simulink model "ADRC_playground"  (R2024b)
settings: Solver=FixedStepAuto  StartTime=0.0  StopTime=10.0  FixedStep=h  RelTol=1e-5
values from neighbouring files (symbols this model uses):
  a1 = 2    [ADRC_playground.m]    (also in ADRC_playground_vars.m)
  a2 = 3    [ADRC_playground.m]    (also in ADRC_playground_vars.m)
  b = 0.2    [ADRC_playground_vars.m]    (also in LADRC_ct_vars.m = [zeros(N-1, 1))
  b0 = 0.4    [ADRC_playground_vars.m]    (also in LADRC_ct_vars.m = 0.75)
  beta1 = 1    [ADRC_playground_vars.m]
  beta2 = 1 / (2*h^0.5)    (= 5)    [ADRC_playground_vars.m]
  beta3 = 2 / (5^2 * h^1.2)    (= 20.0950914521)    [ADRC_playground_vars.m]
  c = 1    [ADRC_playground_vars.m]
  h = 0.01    [ADRC_playground_vars.m]
  r = 5    [ADRC_playground_vars.m]
undefined symbols (not defined in the file or in its folder): DiscIntNeverNeededParam
settings Model: Creator=Henrik  LastModifiedBy=Henrik

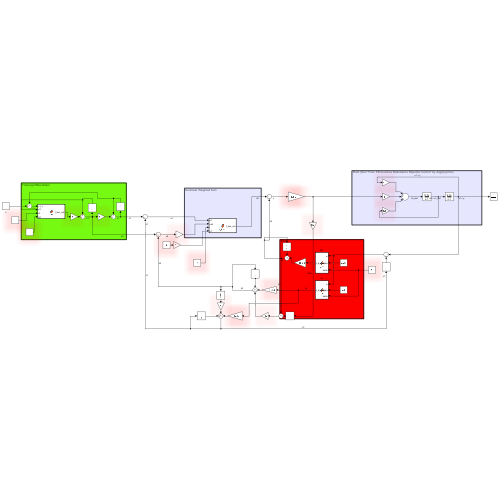
[thumbnail: Simulink's stored preview of the top-level diagram]
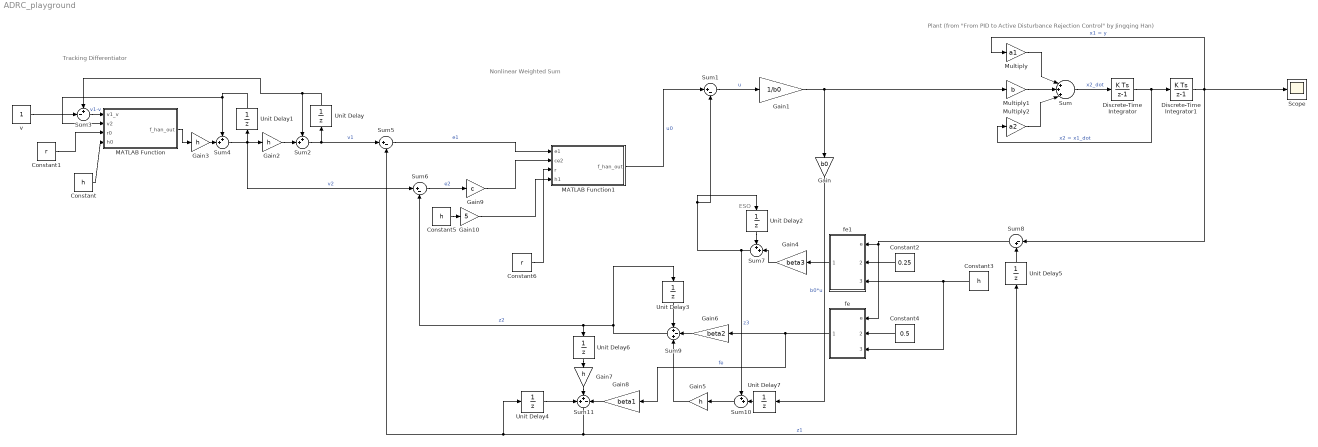
== system ADRC_playground ==
  note: Tracking Differentiator
  note: Nonlinear Weighted Sum
  note: ESO
  note: Plant (from "From PID to Active Disturbance Rejection Control" by Jingqing Han)
  Constant : Constant  Value=h
  Constant1 : Constant  Value=r
  Constant2 : Constant  Value=0.25
  Constant3 : Constant  Value=h
  Constant4 : Constant  Value=0.5
  Constant5 : Constant  Value=h
  Constant6 : Constant  Value=r
  Discrete-Time Integrator : DiscreteIntegrator  SampleTime=-1  ICPrevOutput=DiscIntNeverNeededParam  ICPrevScaledInput=DiscIntNeverNeededParam
  Discrete-Time Integrator1 : DiscreteIntegrator  SampleTime=-1  ICPrevOutput=DiscIntNeverNeededParam  ICPrevScaledInput=DiscIntNeverNeededParam
  Gain : Gain  Gain=b0
  Gain1 : Gain  Gain=1/b0
  Gain10 : Gain  Gain=5
  Gain{2..3,5,7} (4 alike) : Gain  Gain=h
  Gain4 : Gain  Gain=beta3
  Gain6 : Gain  Gain=beta2
  Gain8 : Gain  Gain=beta1
  Gain9 : Gain  Gain=c
  MATLAB Function : MATLAB Function  TreatAsAtomicUnit=on
  MATLAB Function1 : MATLAB Function  TreatAsAtomicUnit=on
  Multiply : Gain  Gain=a1
  Multiply1 : Gain  Gain=b
  Multiply2 : Gain  Gain=a2
  Scope : Scope
  Sum : Sum  Inputs=|+++|
  Sum1 : Sum  Inputs=|+-
  Sum{2,4,7,10} (4 alike) : Sum  Inputs=++|
  Sum11 : Sum  Inputs=++-
  Sum3 : Sum  Inputs=+-|
  Sum5 : Sum  Inputs=|+-
  Sum6 : Sum  Inputs=|+-
  Sum8 : Sum  Inputs=|-+
  Sum9 : Sum  Inputs=+-+
  Unit Delay{,1..7} (8 alike) : UnitDelay  SampleTime=-1  HasFrameUpgradeWarning=on
  fe : MATLAB Function  TreatAsAtomicUnit=on
  fe1 : MATLAB Function  TreatAsAtomicUnit=on
  v : Constant
  wires:
  Multiply2/1 -> Sum/3
  Multiply1/1 -> Sum/2
  Multiply/1 -> Sum/1
  Sum/1 -> Discrete-Time Integrator/1  "x2_dot"
  Discrete-Time Integrator/1 -> Discrete-Time Integrator1/1, Multiply2/1  "x2 = x1_dot"
  Discrete-Time Integrator1/1 -> Scope/1, Sum8/1, Multiply/1  "x1 = y"
  Sum1/1 -> Gain1/1  "u"
  Gain/1 -> Unit Delay7/1  "b0*u"
  Gain1/1 -> Multiply1/1, Gain/1
  Sum7/1 -> Unit Delay2/1, Sum1/2, Sum10/1  "z3"
  MATLAB Function1/1(f_han_out) -> Sum1/1  "u0"
  v/1 -> Sum3/2
  Sum3/1 -> MATLAB Function/1(v1_v)  "v1-v"
  Sum2/1 -> Sum5/1, Unit Delay/1  "v1"
  Unit Delay/1 -> Sum3/1, Sum2/1
  Constant/1 -> MATLAB Function/4(h0)
  Sum4/1 -> Sum6/1, Gain2/1, Unit Delay1/1  "v2"
  Gain2/1 -> Sum2/2
  Unit Delay1/1 -> MATLAB Function/2(v2), Sum4/1
  Gain3/1 -> Sum4/2
  MATLAB Function/1(f_han_out) -> Gain3/1
  Constant1/1 -> MATLAB Function/3(r0)
  Sum9/1 -> Unit Delay6/1, Sum6/2, Unit Delay3/1  "z2"
  fe1/1(f_al_out) -> Gain4/1
  Gain4/1 -> Sum7/2
  Unit Delay2/1 -> Sum7/1
  Sum5/1 -> MATLAB Function1/1(e1)  "e1"
  Sum8/1 -> fe1/1(e), fe/1(e)
  Constant2/1 -> fe1/2(alpha)
  Constant3/1 -> fe1/3(delta), fe/3(delta)
  Unit Delay3/1 -> Sum9/1
  Constant4/1 -> fe/2(alpha)
  fe/1(f_al_out) -> Gain8/1, Gain6/1  "fe"
  Gain6/1 -> Sum9/2
  Sum10/1 -> Gain5/1
  Gain5/1 -> Sum9/3
  Unit Delay4/1 -> Sum11/1
  Sum11/1 -> Unit Delay5/1, Sum5/2, Unit Delay4/1  "z1"
  Gain7/1 -> Sum11/2
  Gain8/1 -> Sum11/3
  Sum6/1 -> Gain9/1  "e2"
  Gain9/1 -> MATLAB Function1/2(ce2)
  Constant5/1 -> Gain10/1
  Gain10/1 -> MATLAB Function1/4(h1)
  Constant6/1 -> MATLAB Function1/3(r)
  Unit Delay5/1 -> Sum8/2
  Unit Delay6/1 -> Gain7/1
  Unit Delay7/1 -> Sum10/2

== matlab function ADRC_playground/fe1 ==
  data: e input; f_al_out output; alpha input; delta input
function f_al_out = f_al(e, alpha, delta)

f_al_out = 0;

if abs(e) <= delta

    f_al_out = e / (delta^(1-alpha));

end 

if abs(e) >= delta

    f_al_out = abs(e)^alpha * sign(e);

end

== matlab function ADRC_playground/MATLAB Function ==
  data: v1_v input; f_han_out output; v2 input; r0 input; h0 input
function f_han_out = f_v(v1_v, v2, r0, h0)

d = h0*r0^2;
a0 = h0*v2;
y = v1_v + a0;

a1 = sqrt(d*(d + 8 * abs(y)));
a2 = a0 + sign(y)*(a1-d)/2;

s_y = (sign(y+d) - sign(y-d)) / 2;

a = (a0 + y - a2)*s_y + a2;
s_a = (sign(a+d) - sign(a*d)) / 2;

f_han_out = -r0 * (a/d * sign(a)) * s_a * r0 * sign(a);

== matlab function ADRC_playground/fe ==
  data: e input; f_al_out output; alpha input; delta input
function f_al_out = f_al(e, alpha, delta)

f_al_out = 0;

if abs(e) <= delta

    f_al_out = e / (delta^(1-alpha));

end 

if abs(e) >= delta

    f_al_out = abs(e)^alpha * sign(e);

end

== matlab function ADRC_playground/MATLAB Function1 ==
  data: e1 input; f_han_out output; ce2 input; r input; h1 input
function f_han_out = f_han(e1, ce2, r, h1)

d = h1*r^2;
a0 = h1*ce2;
y = e1 + a0;

a1 = sqrt(d*(d + 8 * abs(y)));
a2 = a0 + sign(y)*(a1-d)/2;

s_y = (sign(y+d) - sign(y-d)) / 2;

a = (a0 + y - a2)*s_y + a2;
s_a = (sign(a+d) - sign(a*d)) / 2;

f_han_out = -r * (a/d * sign(a)) * s_a * r * sign(a);
